simulink model "lab13"  (R2024a)
settings: Solver=VariableStepAuto  StartTime=0.0  StopTime=100.0  RelTol=1e-3
undefined symbols (not defined in the file): m, n
libraries: simulink x2, dspstat3 x1
settings Model: Creator=user  LastModifiedBy=user
settings OptimizationCC: ReuseModelBlockBuffer=off
settings RTWCC: GPUComputeCapability=3.5

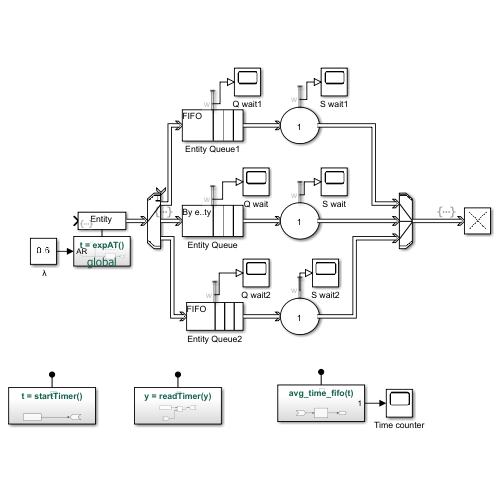
[thumbnail: Simulink's stored preview of the top-level diagram]
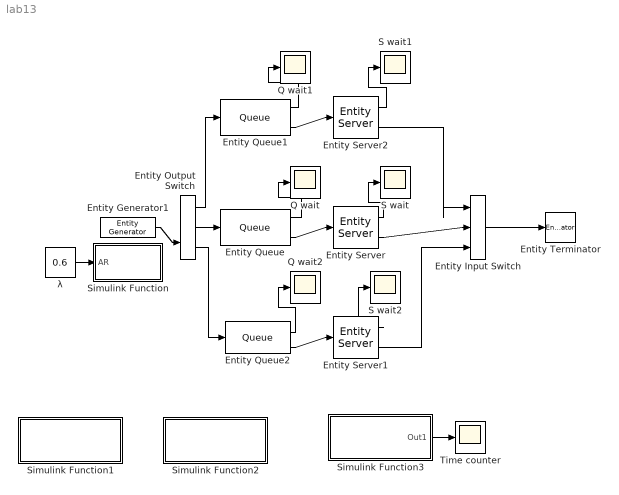
== system lab13 ==
  " λ" : Constant  Value=0.6  SampleTime=-1
  Entity Input Switch : EntityInputSwitch  InputPortMessageModes=m,m,m  OutputPortMessageModes=m  NumberInputPorts=3
      settings: InputPortMap=u1,u2,u3
  Entity Output Switch : EntityOutputSwitch  InputPortMessageModes=m,m  OutputPortMessageModes=m,m,m  NumberOutputPorts=3  SwitchingCriterion=From control port  SwitchAttributeName=Attribute1  InitialPortSelection=3
      settings: InputPortMap=u0,u1  OutputPortMap=o0,o1,o2
  Entity Generator1 : EntityGenerator  OutputPortMessageModes=m  TimeSource=Signal port  IntergenerationTimeAction=dt = expAT();  GenerateAction=|  AttributeName=ServiceTime|Timer  AttributeInitialValue=0|0  EntityType=Structured  EntityTypeName=Entity
      | entity.ServiceTime = exprnd(3);
      | entitySys.priority = randi(2);
      | entity.Timer = 0; % Инициализация Timer
      | entity.Timer = startTimer(); % Запуск таймера
      settings: InputPortMap=u1
  Entity Queue : Queue  InputPortMessageModes=m  OutputPortMessageModes=n,m  Capacity=5  QueueType=Priority  PrioritySource=entitySys.priority  EntryAction=entity.Timer = startTimer();  AverageWait=on
      settings: OutputPortMap=o2,o5
  Entity Queue1 : Queue  InputPortMessageModes=m  OutputPortMessageModes=n,m  Capacity=5  AverageWait=on
      settings: OutputPortMap=o2,o5
  Entity Queue2 : Queue  InputPortMessageModes=m  OutputPortMessageModes=n,m  Capacity=35  PrioritySource=entitySys.priority  AverageWait=on
      settings: OutputPortMap=o2,o5
  Entity Server : EntityServer  InputPortMessageModes=m  OutputPortMessageModes=n,m  Capacity=1  ServiceTimeSource=Attribute  AverageWait=on
      settings: OutputPortMap=o4,o9
  Entity Server1 : EntityServer  InputPortMessageModes=m  OutputPortMessageModes=n,m  Capacity=1  AverageWait=on
      settings: OutputPortMap=o4,o9
  Entity Server2 : EntityServer  InputPortMessageModes=m  OutputPortMessageModes=n,m  Capacity=1  AverageWait=on
      settings: OutputPortMap=o4,o9
  Entity Terminator : EntityTerminator  InputPortMessageModes=m  EntryAction=|
      | elapsedTime = readTimer(entity.Timer);
      | avg_time_fifo(elapsedTime);
  Q wait : Scope
  Q wait1 : Scope
  Q wait2 : Scope
  S wait : Scope
  S wait1 : Scope
  S wait2 : Scope
  Simulink Function : Subsystem  TreatAsAtomicUnit=on
      settings: LibrarySourceBlock=sldelib/Simulink Function
  Simulink Function1 : Subsystem  TreatAsAtomicUnit=on
  Simulink Function2 : Subsystem  TreatAsAtomicUnit=on
  Simulink Function3 : Subsystem  TreatAsAtomicUnit=on
  Time counter : Scope
  wires:
  " λ"/1 -> Simulink Function/1(AR)
  Entity Generator1/1 -> Entity Output Switch/2
  Simulink Function3/1(Out1) -> Time counter/1
  Entity Queue/1 -> Q wait/1
  Entity Queue/2 -> Entity Server/1
  Entity Server/1 -> S wait/1
  Entity Server/2 -> Entity Input Switch/2
  Entity Output Switch/2 -> Entity Queue/1
  Entity Input Switch/1 -> Entity Terminator/1
  Entity Output Switch/3 -> Entity Queue2/1
  Entity Output Switch/1 -> Entity Queue1/1
  Entity Queue1/2 -> Entity Server2/1
  Entity Queue2/2 -> Entity Server1/1
  Entity Server1/2 -> Entity Input Switch/3
  Entity Server2/2 -> Entity Input Switch/1
  Entity Server2/1 -> S wait1/1
  Entity Queue1/1 -> Q wait1/1
  Entity Server1/1 -> S wait2/1
  Entity Queue2/1 -> Q wait2/1

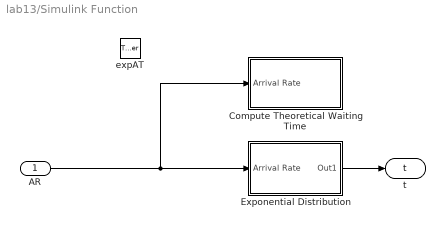
== system lab13/Simulink Function ==
  AR : Inport
  expAT : TriggerPort  TriggerType=function-call  IsSimulinkFunction=on  FunctionName=expAT  VariantControl=Variant
  Compute Theoretical Waiting Time : Subsystem
  Exponential Distribution : Subsystem
  t : ArgOut  DisableCoverage=on  ArgumentName=t
  wires:
  Exponential Distribution/1(Out1) -> t/1
  AR/1 -> Compute Theoretical Waiting Time/1(Arrival Rate), Exponential Distribution/1(Arrival Rate)

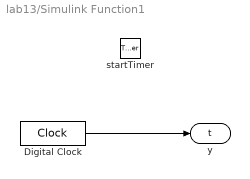
== system lab13/Simulink Function1 ==
  startTimer : TriggerPort  TriggerType=function-call  IsSimulinkFunction=on  FunctionName=startTimer  FunctionVisibility=scoped  VariantControl=(inherit)
  Digital Clock : DigitalClock  SampleTime=-1
  y : ArgOut  DisableCoverage=on  ArgumentName=t
  wires:
  Digital Clock/1 -> y/1

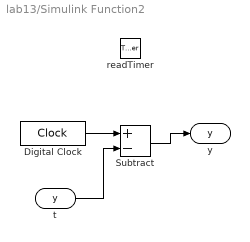
== system lab13/Simulink Function2 ==
  readTimer : TriggerPort  TriggerType=function-call  IsSimulinkFunction=on  FunctionName=readTimer  FunctionVisibility=scoped  VariantControl=(inherit)
  Digital Clock : DigitalClock  SampleTime=-1
  Subtract : Sum  Inputs=+-
  t : ArgIn  DisableCoverage=on  ArgumentName=y
  y : ArgOut  DisableCoverage=on  ArgumentName=y
  wires:
  Digital Clock/1 -> Subtract/1
  t/1 -> Subtract/2
  Subtract/1 -> y/1

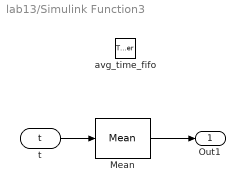
== system lab13/Simulink Function3 ==
  avg_time_fifo : TriggerPort  TriggerType=function-call  IsSimulinkFunction=on  FunctionName=avg_time_fifo  FunctionVisibility=scoped  VariantControl=(inherit)
  Mean : dspstat3/Mean  run=off  InputProcessing=Columns as channels (frame based)  reset_popup=None  directionMode=Each column  dimension=1  roiEnable=off  roiType=Rectangles  roiPortion=Entire ROI  roiOutput=Individual statistics for each ROI  roiFlag=off  roundingMode=Floor  overflowMode=off  outputDataTypeStr=Inherit: Same as accumulator  outputMin=[]  outputMax=[]  outputLastDataTypeStr=Inherit: Same as accumulator
  t : ArgIn  DisableCoverage=on  ArgumentName=t
  Out1 : Outport
  wires:
  Mean/1 -> Out1/1
  t/1 -> Mean/1

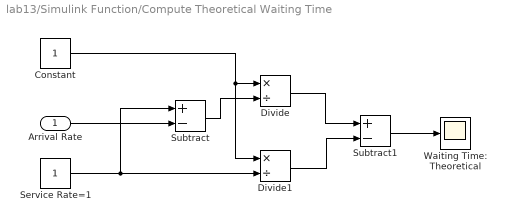
== system lab13/Simulink Function/Compute Theoretical Waiting Time ==
  Arrival Rate : Inport
  Constant : Constant
  Divide : Product  Inputs=*/
  Divide1 : Product  Inputs=*/
  Service Rate=1 : Constant
  Subtract : Sum  Inputs=+-
  Subtract1 : Sum  Inputs=+-
  Waiting Time: Theoretical : Scope
  wires:
  Arrival Rate/1 -> Subtract/2
  Subtract1/1 -> Waiting Time: Theoretical/1
  Divide1/1 -> Subtract1/2
  Divide/1 -> Subtract1/1
  Subtract/1 -> Divide/2
  Constant/1 -> Divide1/1, Divide/1
  Service Rate=1/1 -> Subtract/1, Divide1/2

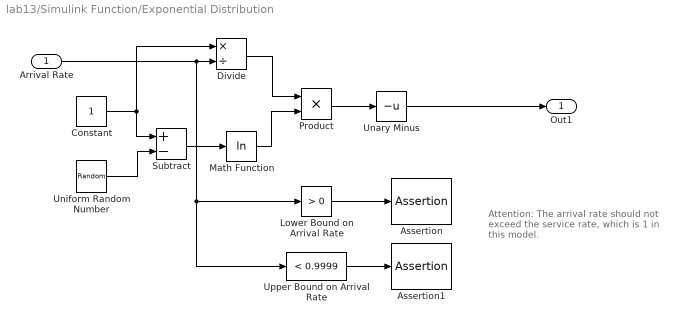
== system lab13/Simulink Function/Exponential Distribution ==
  note: Attention: The arrival rate
      | should not exceed the service
      | rate, which is 1 in this model.
  Arrival Rate : Inport
  Assertion : Assertion
  Assertion1 : Assertion
  Constant : Constant
  Divide : Product  Inputs=*/
  Lower Bound on Arrival Rate : simulink/Logic and Bit Operations/Compare To Constant  relop=>  const=0  OutDataTypeStr=uint8  ZeroCross=off
  Math Function : Math  Operator=log  SignedPower=on
  Product : Product  RndMeth=Zero
  Subtract : Sum  Inputs=+-
  Unary Minus : UnaryMinus
  Uniform Random Number : UniformRandomNumber  Minimum=0  Seed=12345
  "Upper Bound on Arrival Rate " : simulink/Logic and Bit Operations/Compare To Constant  relop=<  const=0.9999  OutDataTypeStr=uint8  ZeroCross=off
  Out1 : Outport
  wires:
  Arrival Rate/1 -> Divide/2, Lower Bound on Arrival Rate/1, "Upper Bound on Arrival Rate "/1
  Unary Minus/1 -> Out1/1
  Product/1 -> Unary Minus/1
  Math Function/1 -> Product/2
  Divide/1 -> Product/1
  Constant/1 -> Divide/1, Subtract/1
  Uniform Random Number/1 -> Subtract/2
  Lower Bound on Arrival Rate/1 -> Assertion/1
  "Upper Bound on Arrival Rate "/1 -> Assertion1/1
  Subtract/1 -> Math Function/1
